simulink model "mod_double_pend"  (R2021a)
settings: Solver=FixedStepAuto  StartTime=0.0  StopTime=10  FixedStep=.01  RelTol=1e-3
model workspace (MAT data in the model file):
  exo_pos_cost_10 : param.Continuous (value not decoded)
values from neighbouring files (symbols this model uses):
  alpha = [15,15]    [play.m]    (also in play_all_cost_parameters.m = params.all_cost_parameters(5,1).Value; play_pos_cost_parameters.m = params.pos_cost_parameters(5,1).Value; play_vel_cost_parameters.m = params.vel_cost_parameters(5,1).Value)
  beta = [ 1/8 ; 1/8]    [play.m]    (also in play_all_cost_parameters.m = params.all_cost_parameters(6,1).Value; play_pos_cost_parameters.m = params.pos_cost_parameters(6,1).Value; play_vel_cost_parameters.m = params.vel_cost_parameters(6,1).Value)
  Bn0 = [500  500]    [play.m]    (also in play_all_cost_parameters.m = params.all_cost_parameters(1,1).Value; play_pos_cost_parameters.m = params.pos_cost_parameters(1,1).Value; play_vel_cost_parameters.m = params.vel_cost_parameters(1,1).Value)
  Bp0 = [500  500]    [play.m]    (also in play_all_cost_parameters.m = params.all_cost_parameters(2,1).Value; play_pos_cost_parameters.m = params.pos_cost_parameters(2,1).Value; play_vel_cost_parameters.m = params.vel_cost_parameters(2,1).Value)
  dampener = [1000, 0; 0, 1000]    [play.m]    (also in play_all_cost_parameters.m; play_pos_cost_parameters.m; play_vel_cost_parameters.m)
  Dm1 = [496.569821348200,0;0,100]    [play.m]    (also in play_all_cost_parameters.m; play_pos_cost_parameters.m; play_vel_cost_parameters.m)
  exo_sat = 150    [play.m]    (also in play_all_cost_parameters.m; play_pos_cost_parameters.m; play_vel_cost_parameters.m)
  gamma = [15,15]    [play.m]    (also in play_all_cost_parameters.m = params.all_cost_parameters(7,1).Value; play_pos_cost_parameters.m = params.pos_cost_parameters(7,1).Value; play_vel_cost_parameters.m = params.vel_cost_parameters(7,1).Value)
  human_sat = 30    [play.m]    (also in play_all_cost_parameters.m = 150; play_pos_cost_parameters.m; play_vel_cost_parameters.m)
  Ked = [ 50, 0; 0, 50]    [play.m]    (also in play_all_cost_parameters.m; play_pos_cost_parameters.m; play_vel_cost_parameters.m)
  Kem = [ 50, 0; 0, 50]    [play.m]    (also in play_all_cost_parameters.m; play_pos_cost_parameters.m; play_vel_cost_parameters.m)
  Km1 = [6017.73151361233,0;0,2898.16820260871]    [play.m]    (also in play_all_cost_parameters.m; play_pos_cost_parameters.m; play_vel_cost_parameters.m)
  Kn0 = [500  500]    [play.m]    (also in play_all_cost_parameters.m = params.all_cost_parameters(3,1).Value; play_pos_cost_parameters.m = params.pos_cost_parameters(3,1).Value; play_vel_cost_parameters.m = params.vel_cost_parameters(3,1).Value)
  Kp0 = [500 500]    [play.m]    (also in play_all_cost_parameters.m = params.all_cost_parameters(4,1).Value; play_pos_cost_parameters.m = params.pos_cost_parameters(4,1).Value; play_vel_cost_parameters.m = params.vel_cost_parameters(4,1).Value)
  lambda2 = [1.2, 0; 0 1.25]    [play.m]    (also in play_all_cost_parameters.m = params.all_cost_parameters(9,1).Value; play_pos_cost_parameters.m = params.pos_cost_parameters(9,1).Value; play_vel_cost_parameters.m = params.vel_cost_parameters(9,1).Value)
  le = [0.324, 0.3900]    [play.m]    (also in play_all_cost_parameters.m = lh; play_pos_cost_parameters.m; play_vel_cost_parameters.m)
  lh = [0.324, 0.3900]    [play.m]    (also in play_all_cost_parameters.m; play_pos_cost_parameters.m; play_vel_cost_parameters.m)
  Md = [10.0, 0; 0, 10.0]    [play.m]    (also in play_all_cost_parameters.m; play_pos_cost_parameters.m; play_vel_cost_parameters.m)
  me = [ 2.11, 1.28]  + mh    [play.m]    (also in play_all_cost_parameters.m; play_pos_cost_parameters.m; play_vel_cost_parameters.m)
  mh = [11.824, 3.848]    [play.m]    (also in play_all_cost_parameters.m; play_pos_cost_parameters.m; play_vel_cost_parameters.m)
  rho2 = [100, 0; 0, 450]    [play.m]    (also in play_all_cost_parameters.m = params.all_cost_parameters(8,1).Value; play_pos_cost_parameters.m = params.pos_cost_parameters(8,1).Value; play_vel_cost_parameters.m = params.vel_cost_parameters(8,1).Value)
  spring = [2000, 0; 0, 2000]    [play.m]    (also in play_all_cost_parameters.m; play_pos_cost_parameters.m; play_vel_cost_parameters.m)
undefined symbols (not defined in the file or in its folder): l, l1, l2, me2
libraries: simulink x4, sharedTrackingLibrary x1, robotcorelib x1
(part 2 of 2)

== matlab function mod_double_pend/addmittance2/MATLAB Function ==
  data: Tid input; K output; Th input; qd input; B output
function [K,B] = fcn(Tid, Th, qd)

Kp0 = [75 0; 0 25];
Kn0 = [50 0; 0 50];
Bp0 = [75 0; 0 25];
Bn0 = [50 0; 0 50];
beta_p = 3;
beta_n = 3;
alpha_p = 0.5;
alpha_n = 0.5;

intention = sign(Th) == sign(qd);
change = abs(Th/Tid);

K = eye(size(intention,1));
B = eye(size(intention,1));
count = 1;
my_intention = [0;0];


for ii =  1:length(intention)
   if intention(ii)
        K(count,count) = Kp0(count,count) + beta_p*change(count);
        B(count,count) = Bp0(count,count) + alpha_p*change(count);
   else
       K(count,count) = Kn0(count,count) - beta_n*change(count);
       B(count,count) = Bn0(count,count) - alpha_n*change(count);
   end
   my_intention(count) = 0;
   count= count + 1;
   

end


end
